simulink model "setup_xplane_R2011b"  (Simulink 8.4)
settings: Solver=ode45  StartTime=0.0  StopTime=10  RelTol=1e-3
libraries: etargetslib x1, dspnetwork x1
settings Model: Creator=abdkadma  LastModifiedBy=abdkadma
settings DataIOCC: SignalLoggingSaveFormat=Dataset
settings DebuggingCC: FcnCallInpInsideContextMsg=EnableAllAsWarning

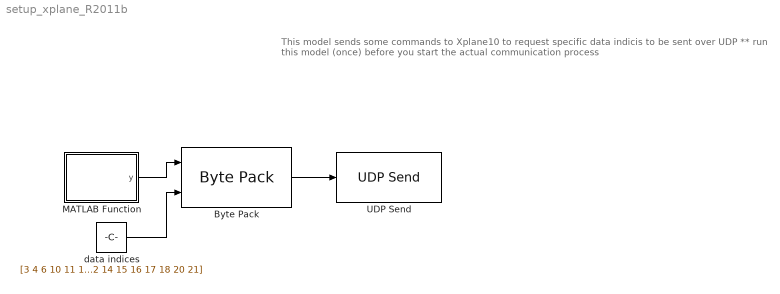
== system setup_xplane_R2011b ==
  note: This model sends some commands to Xplane10
      | to request specific data indicis
      | to be sent over UDP
      | ** run this model (once) before you start the actual communication process
  Byte Pack : etargetslib/Byte Pack  datatypes={'uint8','uint32'}  byteAlign=1
  MATLAB Function : MATLAB Function  TreatAsAtomicUnit=on
  UDP Send : dspnetwork/UDP Send  remoteURL='127.0.0.1'  remotePort=49000  localURL='0.0.0.0'  localPortSource=Automatically determine  localPort=-1  sampletime=-1  separateLengthPort=0
  data indices : Constant  Value=[3 4 6 10 11 12 14 15 16 17 18 20 21]  OutDataTypeStr=uint32
  wires:
  MATLAB Function/1(y) -> Byte Pack/1
  data indices/1 -> Byte Pack/2
  Byte Pack/1 -> UDP Send/1

== matlab function MATLAB Function ==
  data: y output double
function y = fcn()
%#codegen
y = uint8('DSEL0');
